simulink model "DCmotor"  (R2018b)
settings: Solver=FixedStepAuto  StartTime=0.0  StopTime=1.4  FixedStep=0.0002  RelTol=1e-3
values from neighbouring files (symbols this model uses):
  CDtfDen = [0.0021 0.084 0]    [DCmotorSimulationParameters.m]
  DCtfNum = [0.1284]    [DCmotorSimulationParameters.m]
  Kp = PID(1)    [DCmotorSimulationParameters.m]
  Td = PID(3)    [DCmotorSimulationParameters.m]
  Ti = PID(2)    [DCmotorSimulationParameters.m]
settings Model: Creator=root  LastModifiedBy=root

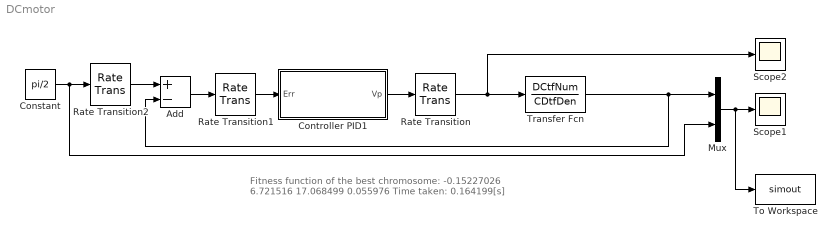
== system DCmotor ==
  note: Fitness function of the best chromosome: -0.15227026
      | 6.721516 17.068499 0.055976
      | Time taken: 0.164199[s]
  Add : Sum  Inputs=+-
  Constant : Constant  Value=pi/2
  Controller PID1 : Subsystem
  Mux : Mux  Inputs=2
  Rate Transition : RateTransition  OutPortSampleTime=0.002
  Rate Transition1 : RateTransition  OutPortSampleTime=0.002
  Rate Transition2 : RateTransition  OutPortSampleTime=0.002
  Scope1 : Scope
  Scope2 : Scope
  To Workspace : ToWorkspace  VariableName=simout  SampleTime=-1
  Transfer Fcn : TransferFcn  Numerator=DCtfNum  Denominator=CDtfDen
  wires:
  Transfer Fcn/1 -> Mux/1, Add/2
  Mux/1 -> To Workspace/1, Scope1/1
  Rate Transition/1 -> Scope2/1, Transfer Fcn/1
  Add/1 -> Rate Transition1/1
  Constant/1 -> Rate Transition2/1, Mux/2
  Rate Transition2/1 -> Add/1
  Rate Transition1/1 -> Controller PID1/1(Err)
  Controller PID1/1(Vp) -> Rate Transition/1

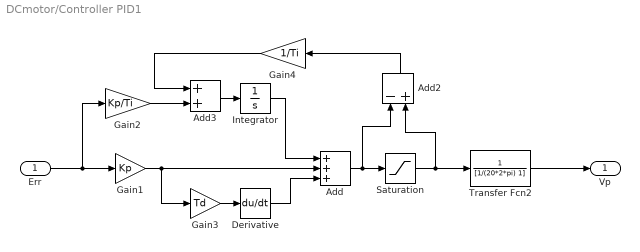
== system DCmotor/Controller PID1 ==
  Err : Inport
  Add : Sum  Inputs=+++
  Add2 : Sum  Inputs=-+
  Add3 : Sum
  Derivative : Derivative
  Gain1 : Gain  Gain=Kp
  Gain2 : Gain  Gain=Kp/Ti
  Gain3 : Gain  Gain=Td
  Gain4 : Gain  Gain=1/Ti
  Integrator : Integrator
  Saturation : Saturate  UpperLimit=10  LowerLimit=-10
  Transfer Fcn2 : TransferFcn  Numerator=1  Denominator=[1/(20*2*pi) 1]
  Vp : Outport
  wires:
  Add2/1 -> Gain4/1
  Add3/1 -> Integrator/1
  Gain2/1 -> Add3/2
  Add/1 -> Saturation/1, Add2/1
  Err/1 -> Gain1/1, Gain2/1
  Integrator/1 -> Add/1
  Gain4/1 -> Add3/1
  Saturation/1 -> Transfer Fcn2/1, Add2/2
  Gain1/1 -> Gain3/1, Add/2
  Transfer Fcn2/1 -> Vp/1
  Derivative/1 -> Add/3
  Gain3/1 -> Derivative/1
